simulink model "QPSK_modulation"  (Simulink 8.1)
settings: Solver=ode45  StartTime=0.0  StopTime=10.0  RelTol=1e-3
undefined symbols (not defined in the file or in its folder): get
libraries: commsink2 x1, commutil2 x1, commrandsrc2 x1
settings Model: Creator=User  LastModifiedBy=Viet
settings DataIOCC: SignalLoggingSaveFormat=Dataset
settings OptimizationCC: ExpressionDepthLimit=128
settings DebuggingCC: FcnCallInpInsideContextMsg=EnableAllAsError
settings GRTTargetCC: CombineOutputUpdateFcns=on  GRTInterface=off

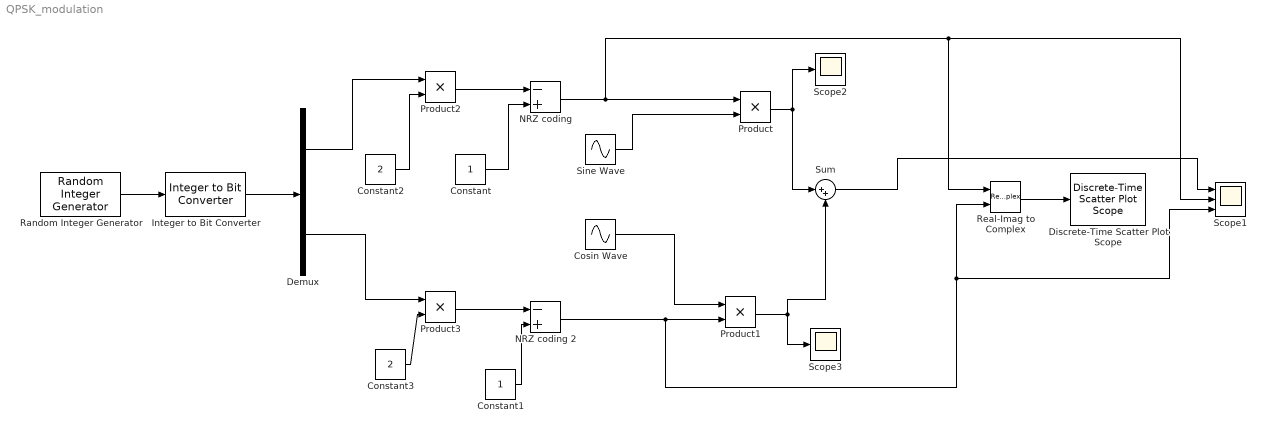
== system QPSK_modulation ==
  Constant : Constant
  Constant1 : Constant
  Constant2 : Constant  Value=2
  Constant3 : Constant  Value=2
  Cosin Wave : Sin  Frequency=20*pi  Phase=pi/2  SampleTime=0.001
  Demux : Demux  Outputs=2
  Discrete-Time Scatter Plot Scope : commsink2/Discrete-Time Scatter Plot Scope  Tag=ScatterPlot  sampPerSymb=1  offsetEye=0  numTraces=40  numNewFrames=40  LineMarkers=*  LineColors=b  fading=on  render=on  AxisGrid=on  xMin=-2  xMax=2  yMin=-2  yMax=2  inphaseLabel=In-phase Amplitude  quadratureLabel=Quadrature Amplitude  openScopeAtSimStart=on  FrameNumber=off  FigPos=get(0,'defaultfigureposition');  figTitle=Scatter Plot  numLinesMax=8  block_type_=scatter
  Integer to Bit Converter : commutil2/Integer to Bit Converter  nbits=2  signedInputValues=Unsigned  bitOrder=MSB first  outDtype=Same as input
  NRZ coding : Sum  Inputs=-+
  NRZ coding 2 : Sum  Inputs=-+
  Product{,1..3} (4 alike) : Product
  Random Integer Generator : commrandsrc2/Random Integer Generator  mul=4  seed=37  Ts=1/10  frameBased=off  sampPerFrame=1  orient=off  outDataType=double
  Real-Imag to Complex : RealImagToComplex
  Scope1 : Scope  NumInputPorts=3
      settings: TimeRange=10  YMin=-2~-2~-2  YMax=2~2~2
  Scope2 : Scope
      settings: YMin=-2  YMax=2  SaveName=ScopeData2
  Scope3 : Scope
      settings: YMin=-2  YMax=2  SaveName=ScopeData3
  Sine Wave : Sin  Frequency=20*pi  SampleTime=0.001
  Sum : Sum  Inputs=|++
  wires:
  Random Integer Generator/1 -> Integer to Bit Converter/1
  Integer to Bit Converter/1 -> Demux/1
  Constant/1 -> NRZ coding/2
  Constant1/1 -> NRZ coding 2/2
  Sum/1 -> Scope1/1
  Constant2/1 -> Product2/2
  Constant3/1 -> Product3/2
  Sine Wave/1 -> Product/2
  Product/1 -> Sum/1, Scope2/1
  Product1/1 -> Sum/2, Scope3/1
  Real-Imag to Complex/1 -> Discrete-Time Scatter Plot Scope/1
  Cosin Wave/1 -> Product1/1
  Demux/1 -> Product2/1
  Product2/1 -> NRZ coding/1
  NRZ coding/1 -> Scope1/2, Real-Imag to Complex/1, Product/1
  Demux/2 -> Product3/1
  Product3/1 -> NRZ coding 2/1
  NRZ coding 2/1 -> Scope1/3, Real-Imag to Complex/2, Product1/2
